simulink model "RobotX_SLAMonly"  (R2014a)
settings: Solver=FixedStepDiscrete  StartTime=0.0  StopTime=inf  FixedStep=.25  RelTol=1e-3
undefined symbols (not defined in the file): Com1, Com2, Com3, Com4, DiscIntNeverNeededParam, standard
libraries: xpcseriallib x11, simulink x3, slrtlib x3, dspmtrx3 x2, speedgoatlib x1, speedgoatlib_IO102 x1
(part 4 of 15)

== matlab function RobotX_SLAMonly/Main FSM/SLAM/Models for prediction/Model43/Non-Holonomic Constraint ==
  data: time input; surgeAccel input; NEyaw output; swayAccel input; YawAccel input; u input; v input; gyrz input; psi input; X input; Y input
function NEyaw  = nonHolonomicNE(time,surgeAccel,swayAccel,YawAccel,u,v,gyrz,psi,X,Y)
%Written by Anderson Lebbad on August 12, 2014
%Last Edited:

%This function estimates the velocities for a new pose based off the 
%velocities and heading calculated from the dynamic model, and the current 
%pose. Uses a non-holonomic constraint for estimation.

%% Find time elapsed for integration

ts = .1;
persistent uPrev vPrev gyrzPrev psiPrev xPrev yPrev

%Initialize
if isempty(uPrev)
    uPrev = [u time];
    vPrev = [v time];
    gyrzPrev = [gyrz time];
    psiPrev = [psi time];
    xPrev = [X time];
    yPrev = [Y time];
end
    
%Update if change
if uPrev(1) ~= u
    uPrev = [u time];
end
if vPrev(1) ~= v
    vPrev = [v time];
end
if gyrzPrev(1) ~= gyrz
    gyrzPrev = [gyrz time];
end
if psiPrev(1) ~= psi
    psiPrev = [psi time];
end
if xPrev(1) ~= X
    xPrev = [X time];
end
if yPrev(1) ~= Y
    yPrev = [Y time];
end

%evaluate elapsed
uTime = ts + time - uPrev(2);
vTime = ts + time - vPrev(2);
gyrzTime = ts + time - gyrzPrev(2);
psiTime = ts + time - psiPrev(2);
xTime = ts + time - xPrev(2);
yTime = ts + time - yPrev(2);

%% Integrate inputs
surgeVel = u + surgeAccel*uTime/2;
swayVel = v + swayAccel*vTime/2;
yawVel = gyrz + YawAccel*gyrzTime/2;
yaw = psi + yawVel*psiTime/2;


%% Apply Non-holonomic constraint for NE velocities
Xd = surgeVel*cos(yaw*pi/180) - swayVel*sin(yaw*pi/180);
Yd = surgeVel*sin(yaw*pi/180) + swayVel*cos(yaw*pi/180);

%% Integrate to output NE coordinates
N = X + Xd*xTime/2;
E = Y + Yd*yTime/2;

NEyaw = [N;E;yaw];

end

== matlab function RobotX_SLAMonly/Main FSM/SLAM/Models for prediction/Model43/move_part ==
  data: PtThrust input; portMP output; PtAzimuth input; StThrust input; StAzimuth input; noiseLevel input; portAzimuth output; stbdMP output; stbdAzimuth output
function [portMP,portAzimuth,stbdMP,stbdAzimuth] = addNoise(PtThrust,...
    PtAzimuth,StThrust,StAzimuth,noiseLevel)
%Written By Anderson Lebbad on September 16, 2014
%Last Edited By:

%This function adds gaussian noise to the inputs for a particular particles
%model

portMP = normrnd(PtThrust, noiseLevel);
portAzimuth = normrnd(PtAzimuth, noiseLevel);
stbdMP = normrnd(StThrust, noiseLevel);
stbdAzimuth = normrnd(StAzimuth, noiseLevel);

end

== matlab function RobotX_SLAMonly/Main FSM/SLAM/Models for prediction/Model44/Dynamic Model ==
  data: F_surge input; F_sway input; Torque input; u input; surgeAccel output; v input; psi input; swayAccel output; yawAccel output
function [surgeAccel, swayAccel, yawAccel] = ...
    WAM_V_3DOF(F_surge, F_sway, Torque, u, v, psi)
%Written by Anderson Lebbad on August 12, 2014
%Last Edited:

%This function was heavily based off of Ariel Qu's Vel3DOF_IvanV1. It was
%rewritten for real-time use.

%This function will produce the transient output surge velocity of a
%linearized model of the USV. It is assumed that the vehicle is equivalent
%to two cylinders in the water.

%%%%%DEFINED VARIABLE%%%%%%
%
%   Xext = Thrust from motors
%   Next = Moment from motor
%   m = Mass of vehicle
%   Xudot = Added mass in surge direction
%   Yvdot = Added mass in sway direction
%   Nrdot = Added mass from yaw
%   xg = offset from center of gravity
%   rho = density of seawater
%   S = wetted surface area
%   R = Reynolds number
%   Cd = Coefficient of drag
%   Cdc = Coefficient of drag for sway
%   nu = Kinematic viscosity
%   L = Length overall
%   T = draft
%   B = beam
%   SA = Surface area of cylinder experiencing sway
%   Iz = moment of inertia about Z axis
%
%%%%%%

% Force/Mometns from thrusters & control surfaces...

tau = [F_surge; F_sway; Torque];

% Calculate yaw rate
persistent lastHeading
if isempty(lastHeading)
    lastHeading = psi;
end
%Sample time
ts = .1;

r = (psi - lastHeading)/ts;

% Velocity & Angular velocity vectors
vel = [u; v; 0];
omega = [0; 0; r];

%define variables
m = 145.7;         % Total mass [kg] - reduced from 102
rho = 1025.9;   % density of seawater [kg/m^3]
L = 3.91*0.85;  % Length on the waterline [m]
B = 0.426;       % Demihull beam [m]
T = B*0.2;        % Draft of the demihull [m]
p_bar = 1.0; % sidehull separation - from centerplane vessel to centerplane demihull
Iz = 262.181;    % Mass moment of inertia about z-axis [kg*m^2]
xg = 0;         % Body-Fixed coordinate system taken to be center of gravity
yg = 0;         % Symmetrical Vessel
Cd = 1.1;       % Drag coefficient for a lateral cylinder
LCG = 1.485;        % Need to know where LCG wrt stern

% Vector location of port and starboard hulls
r_port = [-LCG; -p_bar; 0];   
r_stbd = [-LCG; p_bar; 0];

% Port and starboard hull velocities
vel_port = vel + cross(omega,r_port);
vel_stbd = vel + cross(omega,r_stbd);

u_port = vel_port(1);
u_stbd = vel_stbd(1);

% Port and starboard state vectors
state_port = vel_port + omega;
state_stbd = vel_stbd + omega;

%% Added Mass
% Estimated for each hull, then multiplied by 2 to account for both hulls
Xudot = -0.05*m;

%Using strip theory to estimate added mass coefficients
Nrdot = -(4.75/2*pi*rho*p_bar*T^4 + pi*rho*T^2*((L - LCG)^3 + LCG^3)/3);
Nvdot = - pi*rho*T^2*((L - LCG)^2 - LCG^2)/2;

Yrdot = Nvdot;
Yvdot = -rho*pi*T^2*L;

% Multiply by 2:
Xudot = 2*Xudot;
Nrdot = 2*Nrdot;
Nvdot = 2*Nvdot;
Yrdot = 2*Yrdot;
Yvdot = 2*Yvdot;

%Calculate Coefficient of Drag for Sway from 1950 SNAME approximation
Cdc= 1.1 + 0.0045*L/T - 0.1*B/T + 0.016*(B/T)^2;
SA = 2*pi/4*T*L; %projected area of pontoon for two pontoons

%% Linear Drag Terms
%Total Speed
U = sqrt(u^2+v^2);

Xu = 0;
Yv = -0.5*rho*abs(v)*2*Cdc*SA; %20 was the last working number %from SNAME 1950, x2 for two cylinders
%Nr = -0.5*pi*rho*U*T^2*L^2;
Nr = -pi*rho*U*T^2*L^2*.065;
Nv = -pi*rho*U*T^2*L*.01;
Yr = pi*rho*U*T^2*L*0.2;  %from Newman approximation in Lewandowski

%% Nonlinear Drag Terms

% Drag and Moment due to drag on entire vessel - includes nonlinear and
% linear drag terms
D_port = 0.5*(0.44*u_port^3 - 0.01*u_port^2 + 19*u_port);     % Can assume that this equation also takes into account Xu - so set Xu=0
D_stbd = 0.5*(0.44*u_stbd^3 - 0.01*u_stbd^2 + 19*u_stbd);     % Can assume that this equation also takes into account Xu - so set Xu=0

tau_drag = [-(D_port + D_stbd); 0; (D_stbd - D_port)*p_bar];

Xuu = 0;

%% Maneuvering Coefficient Matrices
% Added Mass Matrix
M = [(m - Xudot)      0              0;...
    0               (m - Yvdot)     (m*xg - Yrdot);...
    0               (m*xg - Nvdot)  (Iz - Nrdot)];

%Centripetal and Added Mass Centripetal force matrices
% C_RB = [
%     0                  0                0
%     0                  0                0
%     0                  0                0
%     ];

% C_RB = [
%     0                  0                -m*(xg*r + v)
%     0                  0                -m*(yg*r - u)
%     m*(xg*r + v)       m*(yg*r - u)     0
%     ];

% C_A = -[ %negative originally
%     0                               0           0
%     0                               0           0
%     0                               0           0
%     ];

% Negating centripetal acceleration for test
C_RB = 0;
C_A = 0;

D = -[Xu  0   0;...
      0   Yv  Yr;...
      0   Nv  Nr];

% Nonlinear Drag Coefficients
D_N = -[Xuu*u   0                       0;...
        0       0                       0;...
        0       0                       0];
    
%% Calculate the port and starboard force vectors
tau_port = -(C_RB + C_A + D + D_N)*state_port;
tau_stbd = -(C_RB + C_A + D + D_N)*state_stbd;


%% Sum the force vectors
tau_tot = tau + tau_drag + tau_port + tau_stbd...
    + cross(r_port,[tau_port(1);tau_port(2);0]) + ...
    cross(r_stbd,[tau_stbd(1);tau_stbd(2);0]);

% Calculate the time derivative of the state vector

accel = M\tau_tot;

%% Separate output

surgeAccel = accel(1);
swayAccel = accel(2);
yawAccel = accel(3);

end

== matlab function RobotX_SLAMonly/Main FSM/SLAM/Models for prediction/Model46/Port Thruster Model ==
  data: portMP input; F_surge output; portAzimuth input; F_sway output; Torque output
function [F_surge,F_sway,Torque]  = PortThruster(portMP,portAzimuth)
%Approximation for Starboard Force and Moment with the input motor power
%and azimuth angle of thruster

%Longitudinal distance from center of mass
longDist =1.007;           %m

%Axial distance from center of mass
axialDist=1.485;            %m

%% Piece-wise thrust calculation

if portMP <= -51.0119
    F = .9140*portMP + 40;
elseif portMP >= 26.8367
    F = 1.658*portMP - 41.01;
else
    F = .12987*portMP;
end

%% Force components
F_surge=F*cos(portAzimuth*pi/180);       %N
F_sway=F*sin(portAzimuth*pi/180);       %N

%% Torque calculation

Torque = F_surge*longDist - F_sway*axialDist;   %N.m

end

== matlab function RobotX_SLAMonly/Main FSM/SLAM/Models for prediction/Model46/Stbd Thruster Model ==
  data: stbdMP input; F_surge output; stbdAzimuth input; F_sway output; Torque output
function [F_surge,F_sway,Torque]  = StarBoardThruster(stbdMP,stbdAzimuth)
%Approximation for Starboard Force and Moment with the input motor power
%and azimuth angle of thruster

%Longitudinal distance from center of mass
longDist =1.007;           %m

%Axial distance from center of mass
axialDist=1.485;            %m

%% Piece-wise thrust calculation

if stbdMP <= -51.0119
    F = .9140*stbdMP + 40;
elseif stbdMP >= 26.8367
    F = 1.658*stbdMP - 41.01;
else
    F = .12987*stbdMP;
end

%% Force components
F_surge=F*cos(stbdAzimuth*pi/180);       %N
F_sway=F*sin(stbdAzimuth*pi/180);       %N

%% Torque calculation

Torque = -F_surge*longDist - F_sway*axialDist;   %N.m

end

== matlab function RobotX_SLAMonly/Main FSM/SLAM/Models for prediction/Model47/Non-Holonomic Constraint ==
  data: time input; surgeAccel input; NEyaw output; swayAccel input; YawAccel input; u input; v input; gyrz input; psi input; X input; Y input
function NEyaw  = nonHolonomicNE(time,surgeAccel,swayAccel,YawAccel,u,v,gyrz,psi,X,Y)
%Written by Anderson Lebbad on August 12, 2014
%Last Edited:

%This function estimates the velocities for a new pose based off the 
%velocities and heading calculated from the dynamic model, and the current 
%pose. Uses a non-holonomic constraint for estimation.

%% Find time elapsed for integration

ts = .1;
persistent uPrev vPrev gyrzPrev psiPrev xPrev yPrev

%Initialize
if isempty(uPrev)
    uPrev = [u time];
    vPrev = [v time];
    gyrzPrev = [gyrz time];
    psiPrev = [psi time];
    xPrev = [X time];
    yPrev = [Y time];
end
    
%Update if change
if uPrev(1) ~= u
    uPrev = [u time];
end
if vPrev(1) ~= v
    vPrev = [v time];
end
if gyrzPrev(1) ~= gyrz
    gyrzPrev = [gyrz time];
end
if psiPrev(1) ~= psi
    psiPrev = [psi time];
end
if xPrev(1) ~= X
    xPrev = [X time];
end
if yPrev(1) ~= Y
    yPrev = [Y time];
end

%evaluate elapsed
uTime = ts + time - uPrev(2);
vTime = ts + time - vPrev(2);
gyrzTime = ts + time - gyrzPrev(2);
psiTime = ts + time - psiPrev(2);
xTime = ts + time - xPrev(2);
yTime = ts + time - yPrev(2);

%% Integrate inputs
surgeVel = u + surgeAccel*uTime/2;
swayVel = v + swayAccel*vTime/2;
yawVel = gyrz + YawAccel*gyrzTime/2;
yaw = psi + yawVel*psiTime/2;


%% Apply Non-holonomic constraint for NE velocities
Xd = surgeVel*cos(yaw*pi/180) - swayVel*sin(yaw*pi/180);
Yd = surgeVel*sin(yaw*pi/180) + swayVel*cos(yaw*pi/180);

%% Integrate to output NE coordinates
N = X + Xd*xTime/2;
E = Y + Yd*yTime/2;

NEyaw = [N;E;yaw];

end

== matlab function RobotX_SLAMonly/Main FSM/SLAM/Models for prediction/Model47/move_part ==
  data: PtThrust input; portMP output; PtAzimuth input; StThrust input; StAzimuth input; noiseLevel input; portAzimuth output; stbdMP output; stbdAzimuth output
function [portMP,portAzimuth,stbdMP,stbdAzimuth] = addNoise(PtThrust,...
    PtAzimuth,StThrust,StAzimuth,noiseLevel)
%Written By Anderson Lebbad on September 16, 2014
%Last Edited By:

%This function adds gaussian noise to the inputs for a particular particles
%model

portMP = normrnd(PtThrust, noiseLevel);
portAzimuth = normrnd(PtAzimuth, noiseLevel);
stbdMP = normrnd(StThrust, noiseLevel);
stbdAzimuth = normrnd(StAzimuth, noiseLevel);

end

== matlab function RobotX_SLAMonly/Main FSM/SLAM/Models for prediction/Model48/Dynamic Model ==
  data: F_surge input; F_sway input; Torque input; u input; surgeAccel output; v input; psi input; swayAccel output; yawAccel output
function [surgeAccel, swayAccel, yawAccel] = ...
    WAM_V_3DOF(F_surge, F_sway, Torque, u, v, psi)
%Written by Anderson Lebbad on August 12, 2014
%Last Edited:

%This function was heavily based off of Ariel Qu's Vel3DOF_IvanV1. It was
%rewritten for real-time use.

%This function will produce the transient output surge velocity of a
%linearized model of the USV. It is assumed that the vehicle is equivalent
%to two cylinders in the water.

%%%%%DEFINED VARIABLE%%%%%%
%
%   Xext = Thrust from motors
%   Next = Moment from motor
%   m = Mass of vehicle
%   Xudot = Added mass in surge direction
%   Yvdot = Added mass in sway direction
%   Nrdot = Added mass from yaw
%   xg = offset from center of gravity
%   rho = density of seawater
%   S = wetted surface area
%   R = Reynolds number
%   Cd = Coefficient of drag
%   Cdc = Coefficient of drag for sway
%   nu = Kinematic viscosity
%   L = Length overall
%   T = draft
%   B = beam
%   SA = Surface area of cylinder experiencing sway
%   Iz = moment of inertia about Z axis
%
%%%%%%

% Force/Mometns from thrusters & control surfaces...

tau = [F_surge; F_sway; Torque];

% Calculate yaw rate
persistent lastHeading
if isempty(lastHeading)
    lastHeading = psi;
end
%Sample time
ts = .1;

r = (psi - lastHeading)/ts;

% Velocity & Angular velocity vectors
vel = [u; v; 0];
omega = [0; 0; r];

%define variables
m = 145.7;         % Total mass [kg] - reduced from 102
rho = 1025.9;   % density of seawater [kg/m^3]
L = 3.91*0.85;  % Length on the waterline [m]
B = 0.426;       % Demihull beam [m]
T = B*0.2;        % Draft of the demihull [m]
p_bar = 1.0; % sidehull separation - from centerplane vessel to centerplane demihull
Iz = 262.181;    % Mass moment of inertia about z-axis [kg*m^2]
xg = 0;         % Body-Fixed coordinate system taken to be center of gravity
yg = 0;         % Symmetrical Vessel
Cd = 1.1;       % Drag coefficient for a lateral cylinder
LCG = 1.485;        % Need to know where LCG wrt stern

% Vector location of port and starboard hulls
r_port = [-LCG; -p_bar; 0];   
r_stbd = [-LCG; p_bar; 0];

% Port and starboard hull velocities
vel_port = vel + cross(omega,r_port);
vel_stbd = vel + cross(omega,r_stbd);

u_port = vel_port(1);
u_stbd = vel_stbd(1);

% Port and starboard state vectors
state_port = vel_port + omega;
state_stbd = vel_stbd + omega;

%% Added Mass
% Estimated for each hull, then multiplied by 2 to account for both hulls
Xudot = -0.05*m;

%Using strip theory to estimate added mass coefficients
Nrdot = -(4.75/2*pi*rho*p_bar*T^4 + pi*rho*T^2*((L - LCG)^3 + LCG^3)/3);
Nvdot = - pi*rho*T^2*((L - LCG)^2 - LCG^2)/2;

Yrdot = Nvdot;
Yvdot = -rho*pi*T^2*L;

% Multiply by 2:
Xudot = 2*Xudot;
Nrdot = 2*Nrdot;
Nvdot = 2*Nvdot;
Yrdot = 2*Yrdot;
Yvdot = 2*Yvdot;

%Calculate Coefficient of Drag for Sway from 1950 SNAME approximation
Cdc= 1.1 + 0.0045*L/T - 0.1*B/T + 0.016*(B/T)^2;
SA = 2*pi/4*T*L; %projected area of pontoon for two pontoons

%% Linear Drag Terms
%Total Speed
U = sqrt(u^2+v^2);

Xu = 0;
Yv = -0.5*rho*abs(v)*2*Cdc*SA; %20 was the last working number %from SNAME 1950, x2 for two cylinders
%Nr = -0.5*pi*rho*U*T^2*L^2;
Nr = -pi*rho*U*T^2*L^2*.065;
Nv = -pi*rho*U*T^2*L*.01;
Yr = pi*rho*U*T^2*L*0.2;  %from Newman approximation in Lewandowski

%% Nonlinear Drag Terms

% Drag and Moment due to drag on entire vessel - includes nonlinear and
% linear drag terms
D_port = 0.5*(0.44*u_port^3 - 0.01*u_port^2 + 19*u_port);     % Can assume that this equation also takes into account Xu - so set Xu=0
D_stbd = 0.5*(0.44*u_stbd^3 - 0.01*u_stbd^2 + 19*u_stbd);     % Can assume that this equation also takes into account Xu - so set Xu=0

tau_drag = [-(D_port + D_stbd); 0; (D_stbd - D_port)*p_bar];

Xuu = 0;

%% Maneuvering Coefficient Matrices
% Added Mass Matrix
M = [(m - Xudot)      0              0;...
    0               (m - Yvdot)     (m*xg - Yrdot);...
    0               (m*xg - Nvdot)  (Iz - Nrdot)];

%Centripetal and Added Mass Centripetal force matrices
% C_RB = [
%     0                  0                0
%     0                  0                0
%     0                  0                0
%     ];

% C_RB = [
%     0                  0                -m*(xg*r + v)
%     0                  0                -m*(yg*r - u)
%     m*(xg*r + v)       m*(yg*r - u)     0
%     ];

% C_A = -[ %negative originally
%     0                               0           0
%     0                               0           0
%     0                               0           0
%     ];

% Negating centripetal acceleration for test
C_RB = 0;
C_A = 0;

D = -[Xu  0   0;...
      0   Yv  Yr;...
      0   Nv  Nr];

% Nonlinear Drag Coefficients
D_N = -[Xuu*u   0                       0;...
        0       0                       0;...
        0       0                       0];
    
%% Calculate the port and starboard force vectors
tau_port = -(C_RB + C_A + D + D_N)*state_port;
tau_stbd = -(C_RB + C_A + D + D_N)*state_stbd;


%% Sum the force vectors
tau_tot = tau + tau_drag + tau_port + tau_stbd...
    + cross(r_port,[tau_port(1);tau_port(2);0]) + ...
    cross(r_stbd,[tau_stbd(1);tau_stbd(2);0]);

% Calculate the time derivative of the state vector

accel = M\tau_tot;

%% Separate output

surgeAccel = accel(1);
swayAccel = accel(2);
yawAccel = accel(3);

end

== matlab function RobotX_SLAMonly/Main FSM/SLAM/Models for prediction/Model50/Port Thruster Model ==
  data: portMP input; F_surge output; portAzimuth input; F_sway output; Torque output
function [F_surge,F_sway,Torque]  = PortThruster(portMP,portAzimuth)
%Approximation for Starboard Force and Moment with the input motor power
%and azimuth angle of thruster

%Longitudinal distance from center of mass
longDist =1.007;           %m

%Axial distance from center of mass
axialDist=1.485;            %m

%% Piece-wise thrust calculation

if portMP <= -51.0119
    F = .9140*portMP + 40;
elseif portMP >= 26.8367
    F = 1.658*portMP - 41.01;
else
    F = .12987*portMP;
end

%% Force components
F_surge=F*cos(portAzimuth*pi/180);       %N
F_sway=F*sin(portAzimuth*pi/180);       %N

%% Torque calculation

Torque = F_surge*longDist - F_sway*axialDist;   %N.m

end

== matlab function RobotX_SLAMonly/Main FSM/SLAM/Models for prediction/Model50/Stbd Thruster Model ==
  data: stbdMP input; F_surge output; stbdAzimuth input; F_sway output; Torque output
function [F_surge,F_sway,Torque]  = StarBoardThruster(stbdMP,stbdAzimuth)
%Approximation for Starboard Force and Moment with the input motor power
%and azimuth angle of thruster

%Longitudinal distance from center of mass
longDist =1.007;           %m

%Axial distance from center of mass
axialDist=1.485;            %m

%% Piece-wise thrust calculation

if stbdMP <= -51.0119
    F = .9140*stbdMP + 40;
elseif stbdMP >= 26.8367
    F = 1.658*stbdMP - 41.01;
else
    F = .12987*stbdMP;
end

%% Force components
F_surge=F*cos(stbdAzimuth*pi/180);       %N
F_sway=F*sin(stbdAzimuth*pi/180);       %N

%% Torque calculation

Torque = -F_surge*longDist - F_sway*axialDist;   %N.m

end

== matlab function RobotX_SLAMonly/Main FSM/SLAM/Landmark Organizer ==
  data: Distances input; lm_data output; Angles input
function lm_data = lmOrganize(Distances,Angles)
%Written By Anderson Lebbad on September 16, 2014
%Last Edited by:

%This function structures the landmark data to be used for the SLAM

landmarks = [0.01*Distances'; pi/180*Angles'];
[M,N] = size(landmarks);
lm_data = landmarks(1:M*N);

end

== matlab function RobotX_SLAMonly/Main FSM/SLAM/Any State Change ==
  data: u input; y output
function y = fcn(u)
%#codegen

y = any(any(u));

end

== matlab function RobotX_SLAMonly/Main FSM/SLAM/Any Landmark Change ==
  data: u input; y output
function y = fcn(u)
%#codegen

y = any(any(u));

end

== matlab function RobotX_SLAMonly/Main FSM/SLAM/Models for prediction/Model1/Non-Holonomic Constraint ==
  data: time input; surgeAccel input; NEyaw output; swayAccel input; YawAccel input; u input; v input; gyrz input; psi input; X input; Y input
function NEyaw  = nonHolonomicNE(time,surgeAccel,swayAccel,YawAccel,u,v,gyrz,psi,X,Y)
%Written by Anderson Lebbad on August 12, 2014
%Last Edited:

%This function estimates the velocities for a new pose based off the 
%velocities and heading calculated from the dynamic model, and the current 
%pose. Uses a non-holonomic constraint for estimation.

%% Find time elapsed for integration

ts = .1;
persistent uPrev vPrev gyrzPrev psiPrev xPrev yPrev

%Initialize
if isempty(uPrev)
    uPrev = [u time];
    vPrev = [v time];
    gyrzPrev = [gyrz time];
    psiPrev = [psi time];
    xPrev = [X time];
    yPrev = [Y time];
end
    
%Update if change
if uPrev(1) ~= u
    uPrev = [u time];
end
if vPrev(1) ~= v
    vPrev = [v time];
end
if gyrzPrev(1) ~= gyrz
    gyrzPrev = [gyrz time];
end
if psiPrev(1) ~= psi
    psiPrev = [psi time];
end
if xPrev(1) ~= X
    xPrev = [X time];
end
if yPrev(1) ~= Y
    yPrev = [Y time];
end

%evaluate elapsed
uTime = ts + time - uPrev(2);
vTime = ts + time - vPrev(2);
gyrzTime = ts + time - gyrzPrev(2);
psiTime = ts + time - psiPrev(2);
xTime = ts + time - xPrev(2);
yTime = ts + time - yPrev(2);

%% Integrate inputs
surgeVel = u + surgeAccel*uTime/2;
swayVel = v + swayAccel*vTime/2;
yawVel = gyrz + YawAccel*gyrzTime/2;
yaw = psi + yawVel*psiTime/2;


%% Apply Non-holonomic constraint for NE velocities
Xd = surgeVel*cos(yaw*pi/180) - swayVel*sin(yaw*pi/180);
Yd = surgeVel*sin(yaw*pi/180) + swayVel*cos(yaw*pi/180);

%% Integrate to output NE coordinates
N = X + Xd*xTime/2;
E = Y + Yd*yTime/2;

NEyaw = [N;E;yaw];

end

== matlab function RobotX_SLAMonly/Main FSM/SLAM/SLAM enabled/slammed ==
  data: mpa output; lm_data input; pre_part_positions input; part_positions output
%% SLAM by Chidananda Matada Shivananda
%  Copyright 2010 Randolph Voorhies

%  Edited 2014 Nick DiLeo - Modifications for unknown data association
%  and multiple measurements in a single timestep

%  Edited 2014 Chidananda Matada Shivananda - Simulink compatability, New
%  clustering technique added

%  This program is free software: you can redistribute it and/or modify
%  it under the terms of the GNU General Public License as published by
%  the Free Software Foundation, either version 3 of the License, or
%  (at your option) any later version.
%
%  This program is distributed in the hope that it will be useful,
%  but WITHOUT ANY WARRANTY; without even the implied warranty of
%  MERCHANTABILITY or FITNESS FOR A PARTICULAR PURPOSE.  See the
%  GNU General Public License for more details.
%
%  You should have received a copy of the GNU General Public License
%  along with this program.  If not, see <http://www.gnu.org/licenses/>.

function [mpa,part_positions]   = slammed(lm_data,pre_part_positions)

%% General comments

% the angles in radians
% the ditance in m



%% Initialisations.

persistent particles avg_robot;
num_particles = 50;

% the limits
max_read_distance = 20;
min_read_distance = 0.3;
min_read_angle = -60*pi/180; %radians- maximum read angle
max_read_angle = 60*pi/180;

% The initial starting position of the robot Use UTM coordinates from GPS
avg_robot_position = [0;0;0];% x y rotation

% The Gaussian variance of the movement commands
% Approximating there are only two drives
% movement_variance = [.1;.1];   % Left drive Right_drive
% M = [movement_variance(1), 0.0;
%      0.0, movement_variance(2)];
measurement_variance = [0.01; 0.01];   % Distance Angle
R = [measurement_variance(1), 0.0;
    0.0, measurement_variance(2)];

default_importance=0.00000000001;

if isempty(particles)
    %  Particles
    %             w[1]
    %             position[1,3]
    %             num_landmarks[300] this is to keep history
    
    %             lm_weight[2,15]based on number of landmarks
    %             landmarks[15]
    %                         position[2,1]
    %                         E[2,2]
    %                         counter[1]
    particles=repmat(struct('w',1.0/num_particles,'position',avg_robot_position,'num_landmarks',zeros(1,2),'lm_weight',repmat(1.0/num_particles,2,15),'landmarks',repmat(struct('pos',zeros(1,2),'E',zeros(2,2),'counter',0),1,15)),1,50);
    avg_robot_position = average_pos(particles,num_particles);
end

if isempty(avg_robot)
    avg_robot=avg_robot_position;
end


avg_robot_position=avg_robot;

%% Upload the moved data onto the particles
for shiva9=1:50
    particles(shiva9).position(1)= pre_part_positions(3*(shiva9-1)+1);
    particles(shiva9).position(2)= pre_part_positions(3*(shiva9-1)+1);
    particles(shiva9).position(3)= pre_part_positions(3*(shiva9-1)+1);
end

%% Try to take a reading from each landmark and calculate the Jacobian
doResample = false;
% The input got from landmarks
[~,cols]=find(lm_data ~= 0);
if (isempty(cols)==0)% if the cols is not empty
    doResample=true; %if there is new measurement, then resample particles
end

if (doResample==true)
    [r,~]=size(cols);
    shiva=1;
    G=zeros(2,2,ceil(r/2));
    z_real=zeros(2,ceil(r/2));
    read_distance=zeros(ceil(r/2));
    read_angle=zeros(ceil(r/2));
    
    for lIdx = 1:2:r %amount of visible landmarks
        real_landmark = [lm_data(cols(lIdx+1)),lm_data(cols(lIdx))];
        % Take a real (noisy) measurement from the robot to the landmark
        %         [z_real(:,lIdx), G(:,:,lIdx)] = getRealMeasurement(avg_robot_position, real_landmark, [0 0]);
        %         function [z, H] = getRealMeasurement(pos, landmark_pos, observation_variance)
        
        landmark_angle=real_landmark(1);
        landmark_distance=real_landmark(2);
        % Compute the Jacobian of this measurement function
        q = landmark_distance^2.0;
        G(:,:,shiva) = [-(real_landmark(1) - avg_robot_position(1))/sqrt(q), -(real_landmark(2) - avg_robot_position(2))/sqrt(q);
            (real_landmark(2) - avg_robot_position(2))/q,       -(real_landmark(1) - avg_robot_position(1))/q];
        
        z_real(:,shiva) = [landmark_distance; landmark_angle];
        read_distance(shiva) = z_real(1,shiva);
        read_angle(shiva)    = z_real(2,shiva);
        shiva=shiva+1;
    end
    %     shiva=1;
    
    for pIdx = 1:num_particles
        %     particles(pIdx).lm_weight=[];
        %     clear z_p H Q
        %         coder.varsize('H', [2,2,16],[0 0 1]);
        num_landmarks=particles(pIdx).num_landmarks(1);
        assert(num_landmarks<20);
        H=zeros(2,2,num_landmarks);
        %         coder.varsize('z_p', [2 1 16]);
        z_p=zeros(2,1,num_landmarks);
        Q=zeros(2,2,num_landmarks);
        for j=1:particles(pIdx).num_landmarks(1)
            %             [z_p(:,j), H(:,:,j)] = getMeasurement(particles(pIdx).position, particles(pIdx).landmarks(j).pos, [0 0]);
            %             function [z, H] = getRealMeasurement(pos, landmark_pos, observation_variance)
            landmark_angle=particles(pIdx).landmarks(j).pos(1);
            landmark_distance=particles(pIdx).landmarks(j).pos(2);
            
            % Compute the Jacobian of this measurement function
            q = landmark_distance^2.0;
            %   H = [-(landmark_pos(1) - pos(1))/sqrt(q), -(landmark_pos(2) - pos(2))/sqrt(q), 0.0;
            %         (landmark_pos(2) - pos(2))/q,       -(landmark_pos(1) - pos(1))/q,      -1.0;
            %         0.0,                                0.0,                               1.0];
            
            H(:,:,j) = [-(particles(pIdx).landmarks(j).pos(1) - particles(pIdx).position(1))/sqrt(q), -(particles(pIdx).landmarks(j).pos(2) - particles(pIdx).position(2))/sqrt(q);
                (particles(pIdx).landmarks(j).pos(2) - particles(pIdx).position(2))/q,       -(particles(pIdx).landmarks(j).pos(1) - particles(pIdx).position(1))/q];
            
            
            z_p(:,j) = [landmark_distance;
                landmark_angle];
            
            for measured_lm=1:size(z_real,2)
                residual = z_real(:,measured_lm) - z_p(:,j);
                Q(:,:,j) = H(:,:,j)' * particles(pIdx).landmarks(j).E * H(:,:,j) + R;
                particles(pIdx).lm_weight(measured_lm,j) = particles(pIdx).w * norm(2*pi*Q(:,:,j)).^(-1/2)*exp(-1/2*(residual'/Q(:,:,j)*residual));
            end
        end
        
        particles(pIdx).num_landmarks(2)=particles(pIdx).num_landmarks(1);
        num_landmarks2=particles(pIdx).num_landmarks(2);
        assert(num_landmarks2<20);
        
        %           clear c_hat
        %         clear cost_table data_associate_mat data_associate_vect
        %%%%%%%%%%%%%%%%%%%%%%%%%%%%%%%%%%%%%%%%%%%%%%%%%%%%%%%%%%%%%%%%%%%%%%%%%%%%%%%%%%%%%%%%%%%%%%%%%%%%%%%%%%%%%%%%%%%%%%%%%%%%%%%%%%%%%%%%%%%%%
        cost_table=zeros(size(z_real,2),num_landmarks+size(z_real,2));
        %         cost_table=zeros(size(z_real,2),num_landmarks);
        cost_table(1:size(z_real,2),1:particles(pIdx).num_landmarks(1))=particles(pIdx).lm_weight(1:size(z_real,2),1:particles(pIdx).num_landmarks(1));
        cost_table(1:size(z_real,2),particles(pIdx).num_landmarks(1)+1:particles(pIdx).num_landmarks(1)+size(z_real,2)) =default_importance*eye(size(z_real,2));
        
        particles(pIdx).w=max(max(cost_table,[],1),[],2);
        [~, idx_hold]=max(cost_table,[],1); %this is the max correseponding for each measurement
        for i=1:size(cost_table,2)
            idx_zero=setdiff(1:size(cost_table,1),idx_hold(i));
            cost_table(idx_zero,i)=0;
        end
        
        cost_table1=cost_table;
        for shiva14=1:size(cost_table,2)
            cost_table(:,shiva14)=cost_table1(:,size(cost_table,2)-shiva14+1);
        end
        
        
        new_landmarks=0;
        for measured_lm=1:size(z_real,2)
            [~, IDX] = max(cost_table(measured_lm,:));
            if IDX > particles(pIdx).num_landmarks(1)
                new_landmarks=new_landmarks+1;
            end
        end
        
        
        assert(new_landmarks<20);
        data_associate_mat=zeros(size(z_real,2),new_landmarks+num_landmarks2);
        
        for measured_lm=1:size(z_real,2)
            [~, IDX] = max(cost_table(measured_lm,:));
            if IDX > particles(pIdx).num_landmarks(1)
                %we haven't seen this landmark before
                %                 if particles(pIdx).num_landmarks(2)>14
                %                     break;
                %                 end
                particles(pIdx).num_landmarks(2)=particles(pIdx).num_landmarks(2)+1; %add new landmark
                data_associate_mat(measured_lm,particles(pIdx).num_landmarks(2))=measured_lm; %set correspondance b/t measurement and feature j
            else
                %we've already seen this landmark
                %           [val idx]=max(particles(pIdx).lm_weight(measured_lm,:));
                data_associate_mat(measured_lm,IDX)=measured_lm; %measurement is a known feature
            end
            
        end
        
        num_landmarks2=particles(pIdx).num_landmarks(2);
        assert(num_landmarks2<20);
        Hn=zeros(2,2,num_landmarks2);
        t=size(H);
        for i=1:t(3)
            Hn(:,:,i)=H(:,:,i);
        end
        
        %         H=zeros(2,2,num_landmarks2);
        H=Hn;
        
        data_associate_vect=max(data_associate_mat,[],1); %vector that contains measurement correspondance to landmarks
        i=1;
        feature_to_delete=zeros(num_landmarks2);
        for j=1:particles(pIdx).num_landmarks(2) %length(data_associate_vect)
            if (data_associate_vect(j)>0 && j>particles(pIdx).num_landmarks(1))
                % If we have never seen this landmark, then we need to initialize it.
                % We'll just use whatever first reading we recieved.
                particles(pIdx).landmarks(j).pos = [particles(pIdx).position(1) + ...
                    sin(read_angle(data_associate_vect(j))+particles(pIdx).position(3))*read_distance(data_associate_vect(j));...
                    particles(pIdx).position(2) + cos(read_angle(data_associate_vect(j))+particles(pIdx).position(3))*read_distance(data_associate_vect(j))]';
                % Initialize the landmark position covariance
                H(:,:,j)=G(:,:,data_associate_vect(j));
                particles(pIdx).landmarks(j).E = inv(G(:,:,data_associate_vect(j)))' * R * inv(G(:,:,data_associate_vect(j)));
                particles(pIdx).landmarks(j).counter=1; %initialize counter
            elseif (data_associate_vect(j)>0 && j<=particles(pIdx).num_landmarks(1))
                %we've seen this landmark before
                K = particles(pIdx).landmarks(j).E * H(:,:,j) / Q(:,:,j);
                % Mix the ideal reading, and our actual reading using the Kalman gain, and use the result
                % to predict a new landmark position
                particles(pIdx).landmarks(j).pos = particles(pIdx).landmarks(j).pos + (K*(z_real(:,data_associate_vect(j))-z_p(:,j)))';
                % Update the covariance of this landmark
                particles(pIdx).landmarks(j).E = (eye(size(H(:,:,j))) - K*H(:,:,j)')*particles(pIdx).landmarks(j).E;
                particles(pIdx).landmarks(j).counter=particles(pIdx).landmarks(j).counter+1; %increment counter
            else
                % We are leaving these unchanged.  These are commented
                % out, but this is what is actually happening in alg.
                % particles(pIdx).landmarks(j).pos = particles(pIdx).landmarks(j).pos;
                % particles(pIdx).landmarks(j).E=particles(pIdx).landmarks(j).E;
                dist_to_landmark=norm([particles(pIdx).landmarks(j).pos(1)-particles(pIdx).position(1) particles(pIdx).landmarks(j).pos(2)-particles(pIdx).position(2)]);
                ang_to_landmark=atan2((particles(pIdx).landmarks(j).pos(1) - particles(pIdx).position(1)),...
                    (particles(pIdx).landmarks(j).pos(2) - particles(pIdx).position(2)))-particles(pIdx).position(3);
                if (dist_to_landmark > max_read_distance ||dist_to_landmark < min_read_distance || ang_to_landmark > max_read_angle || ang_to_landmark < min_read_angle)
                    %counter(pIdx,j)=counter(pIdx,j) %don't change counter
                else
                    particles(pIdx).landmarks(j).counter=particles(pIdx).landmarks(j).counter-1; %decrement counter
                    if particles(pIdx).landmarks(j).counter<0
                        feature_to_delete(i)=j; %we're going to delete all these features at the end of the loop
                        i=i+1;
                    end
                end
                %
            end %if
        end %end j
        %     'pos',zeros(1,2),'E',zeros(2,2),'counter',0
        if~(isempty(nonzeros(feature_to_delete)))
            tobe_del=nonzeros(feature_to_delete);
            for shiva4=1:length(feature_to_delete)
                particles(pIdx).landmarks(tobe_del(shiva4)).pos=zeros(1,2);
                particles(pIdx).landmarks(tobe_del(shiva4)).E=zeros(2,2);
                particles(pIdx).landmarks(tobe_del(shiva4)).counter=0;
            end
            particles(pIdx).num_landmarks(2)= particles(pIdx).num_landmarks(2)-length(tobe_del);
        end
        
        particles(pIdx).num_landmarks(1)=particles(pIdx).num_landmarks(2);
        
    end %pIdx
    
    particles=resample(particles) ;
    
    
    
end% if (doResample==true)


%% Clustering
landmarks_positions=zeros(15*50,2);
row_counter=0;
for pIdx=1:num_particles
    for j=1:15 %this should be index timestep when in full script
        row_counter=row_counter+1;
        landmarks_positions(row_counter,:)=particles(pIdx).landmarks(j).pos(1:2)';
    end
end

mpa=cluster(landmarks_positions);


%% Final changes to be persistent
avg_robot=avg_robot_position;
part_positions=zeros(150,1);

for shiva9=1:3:150
    part_positions(shiva9)=particles(ceil(shiva9/3)).position(1);
    part_positions(shiva9+1)=particles(ceil(shiva9/3)).position(2);
    part_positions(shiva9+2)=particles(ceil(shiva9/3)).position(3);
end

%% Display and output

end %function [y,y1]  = slammed(imu_data,lm_data)

function [map]= cluster(data)

n=size(data,1);
clusters=ones(n,1);
hubs=zeros(n,1);
hubs(1,1)=1;
dif=zeros(n,2);
% clustersort=zeros(n,3);
for i = 1:n
    dif(i,:)= data(clusters(i),:) - data(i,:);
end
dist =sum((dif.*dif),2);
counter =1;             %Keeps track of number of the present number of hubs
continue12 = 1;   % 1=true 0=false indicates whether to continue forming new

while continue12
    counter = counter + 1;    % adding new hub
    if counter>750
        break;
    end
    [~,i]=max(dist);        %m= maximum value in the distance array
    %i is the location of the maximum value in the
    % array
    hubs(counter)=i;        %assigns index to new hub
    temp = i*ones(n,1);
    dif1=zeros(n,2);
    for i23 = 1:n
        dif1(i23,:)= data(temp(i23),:) - data(i23,:);
    end
    newdist =sum((dif1.*dif1),2);
    for r=1:n
        if newdist(r) < dist(r)
            dist(r)=newdist(r);
            clusters(r)=i;
        end     %end for if
    end
    maxdist=max(dist);      %returns distance of point farthest from its hub
    continue12 = farout(counter,hubs,data,maxdist); %Checks the stop condition
end
clustersort=[data,clusters];
clustersort=sortrows(clustersort,3);
map=zeros(12,2);
temp=zeros(12,1);
temp(1,1)=clustersort(1,3);
shiva12=1;
for i=1:n
    if sum(temp==clustersort(i,3)) == 0
        shiva12=shiva12+1;
        if shiva12>12
            break
        end
        temp(shiva12)=clustersort(i,3);
    end
end
for shiva13=1:12
    clusterIdx = clustersort(:,3)==temp(shiva13);
    map(shiva13,:)=[sum(clustersort(clusterIdx,1)),sum(clustersort(clusterIdx,2))*180/pi]/sum(clusterIdx);
end
end



function continue1 = farout(counter1,hubs1,data1,maxdist1)

%FAROUT continue = farout(counter,hubs,data,maxdist)
%       Calculates stop condition.  Stops if the point farthest from its
%       hub is within the average distance value.

index1 = 0;
n=size(data1,1);
dif=zeros(n,2);
for i1 = 1:(counter1-1)
    for j = i1+1 : counter1
        index1 = index1 + 1;
        if index1>750
            break
        end
        dif(index1,:)=data1(hubs1(i1),:) - data1(hubs1(j),:);
    end
end

dist=sqrt(sum((dif.*dif),2));
average_dist = sum(dist)/(2*index1);
if sqrt(maxdist1) < average_dist/4
    continue1 = 0;
else continue1 =1;
end
end                             % end for farout

function avg_robot_position = average_pos(particles,num_particles)
xsiva=0;
ysiva=0;
rotasiva=0;

for siva=1:num_particles
    xsiva=xsiva+particles(siva).position(1);
    ysiva=ysiva+particles(siva).position(2);
    rotasiva=rotasiva+particles(siva).position(3);
end

avg_robot_position = [xsiva/num_particles; ysiva/num_particles; rotasiva/num_particles];

end

function [newParticles] = resample(oldParticles)
% Resample a group of particles such that those with higher weights have a
% higher chance of being replicated, and those with low weights have a high
% chance of disappearing
num_particles=50;
avg_robot_position = [0;0;0];% x y rotation
newParticles=repmat(struct('w',1.0/num_particles,'position',avg_robot_position,'num_landmarks',zeros(1,2),'lm_weight',repmat(1.0/num_particles,2,15),'landmarks',repmat(struct('pos',zeros(1,2),'E',zeros(2,2),'counter',0),1,15)),1,50);

weightSum = 0;
for i=1:length(oldParticles)
    weightSum = weightSum + oldParticles(i).w;
end
for i=1:length(oldParticles)
    oldParticles(i).w = oldParticles(i).w/weightSum;
end
M = length(oldParticles);
%   newParticles = [];
r = rand / M;
c = oldParticles(1).w;
i = 1;
shiva6=1;
assert(shiva6<51);
for m=1:M
    U = r + (m-1) * M^(-1);
    while U > c
        i = i+1;
        c = c+oldParticles(i).w;
    end
    newParticles(shiva6) = oldParticles(i);
    shiva6=shiva6+1;
end
for i=1:length(newParticles)
    newParticles(i).w = 1.0/length(newParticles);
end
end

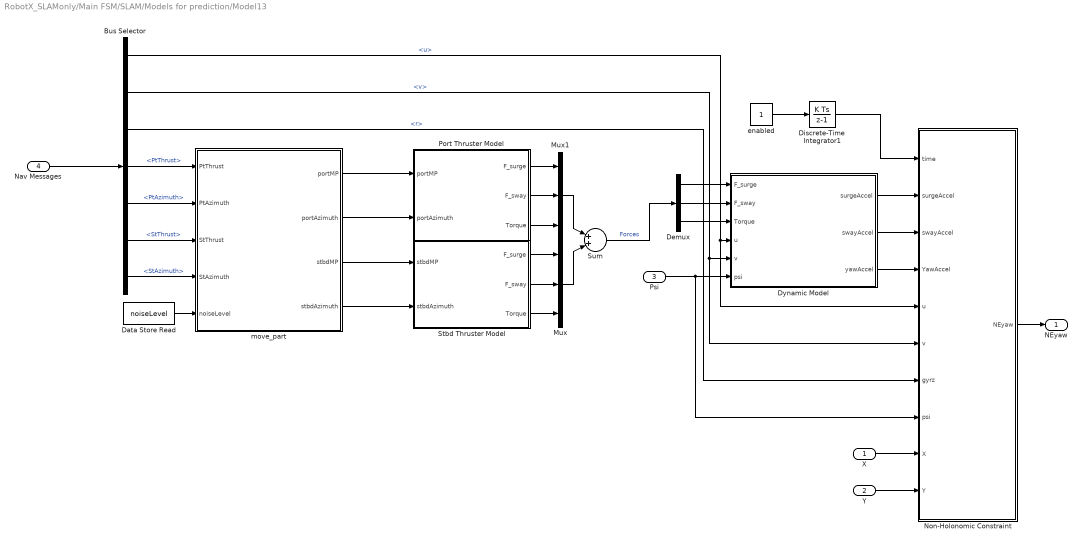
== system RobotX_SLAMonly/Main FSM/SLAM/Models for prediction/Model13 ==
  X : Inport
  Y : Inport  Port=2
  Psi : Inport  Port=3
  Nav Messages : Inport  Port=4
  Bus Selector : BusSelector  OutputSignals=Velocity.u,Velocity.v,Velocity.r,Port.PtThrust,Port.PtAzimuth,Stbd.StThrust,Stbd.StAzimuth
  Data Store Read : DataStoreRead  DataStoreName=noiseLevel
  Demux : Demux  Outputs=3
  Discrete-Time Integrator1 : DiscreteIntegrator  SampleTime=-1  ICPrevOutput=DiscIntNeverNeededParam  ICPrevScaledInput=DiscIntNeverNeededParam
  Dynamic Model : MATLAB Function  TreatAsAtomicUnit=on
  Mux : Mux  Inputs=3
  Mux1 : Mux  Inputs=3
  Non-Holonomic Constraint : MATLAB Function  TreatAsAtomicUnit=on
  Port Thruster Model : MATLAB Function  TreatAsAtomicUnit=on
  Stbd Thruster Model : MATLAB Function  TreatAsAtomicUnit=on
  Sum : Sum  Inputs=|++|
  enabled : Constant
  move_part : MATLAB Function  TreatAsAtomicUnit=on
  NEyaw : Outport
  wires:
  Sum/1 -> Demux/1  "Forces"
  Bus Selector/2 -> Non-Holonomic Constraint/6(v), Dynamic Model/5(v)  "<v>"
  Bus Selector/1 -> Non-Holonomic Constraint/5(u), Dynamic Model/4(u)  "<u>"
  Psi/1 -> Non-Holonomic Constraint/8(psi), Dynamic Model/6(psi)
  Demux/2 -> Dynamic Model/2(F_sway)
  Demux/3 -> Dynamic Model/3(Torque)
  Demux/1 -> Dynamic Model/1(F_surge)
  Mux/1 -> Sum/2
  Stbd Thruster Model/1(F_surge) -> Mux/1
  Stbd Thruster Model/3(Torque) -> Mux/3
  Stbd Thruster Model/2(F_sway) -> Mux/2
  Mux1/1 -> Sum/1
  Port Thruster Model/2(F_sway) -> Mux1/2
  Port Thruster Model/1(F_surge) -> Mux1/1
  Port Thruster Model/3(Torque) -> Mux1/3
  Dynamic Model/1(surgeAccel) -> Non-Holonomic Constraint/2(surgeAccel)
  Dynamic Model/2(swayAccel) -> Non-Holonomic Constraint/3(swayAccel)
  Dynamic Model/3(yawAccel) -> Non-Holonomic Constraint/4(YawAccel)
  Y/1 -> Non-Holonomic Constraint/10(Y)
  X/1 -> Non-Holonomic Constraint/9(X)
  Bus Selector/3 -> Non-Holonomic Constraint/7(gyrz)  "<r>"
  Non-Holonomic Constraint/1(NEyaw) -> NEyaw/1
  enabled/1 -> Discrete-Time Integrator1/1
  Discrete-Time Integrator1/1 -> Non-Holonomic Constraint/1(time)
  Nav Messages/1 -> Bus Selector/1
  Bus Selector/4 -> move_part/1(PtThrust)  "<PtThrust>"
  Bus Selector/5 -> move_part/2(PtAzimuth)  "<PtAzimuth>"
  Bus Selector/7 -> move_part/4(StAzimuth)  "<StAzimuth>"
  Bus Selector/6 -> move_part/3(StThrust)  "<StThrust>"
  move_part/1(portMP) -> Port Thruster Model/1(portMP)
  move_part/2(portAzimuth) -> Port Thruster Model/2(portAzimuth)
  move_part/3(stbdMP) -> Stbd Thruster Model/1(stbdMP)
  move_part/4(stbdAzimuth) -> Stbd Thruster Model/2(stbdAzimuth)
  Data Store Read/1 -> move_part/5(noiseLevel)

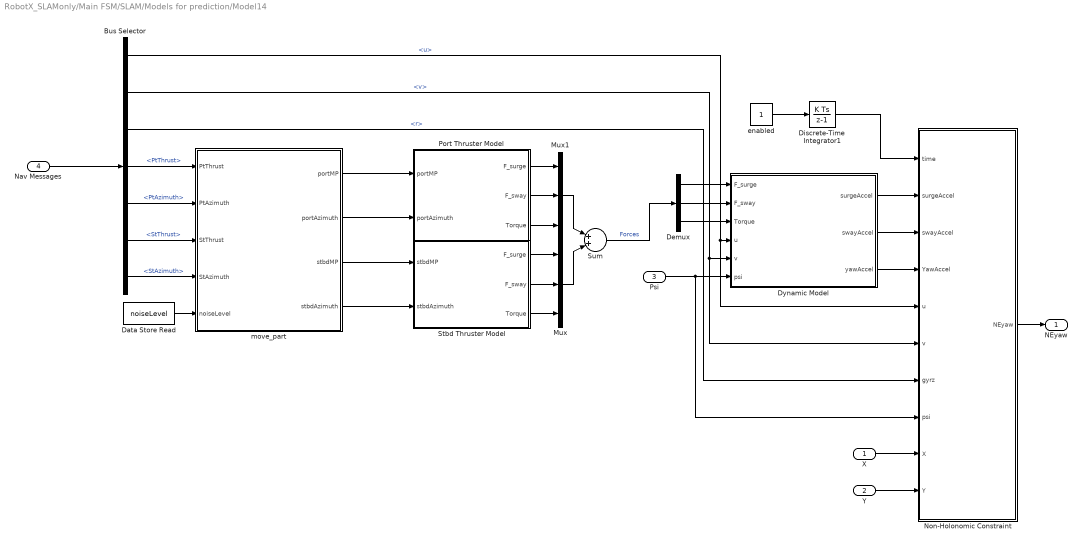
== system RobotX_SLAMonly/Main FSM/SLAM/Models for prediction/Model14 ==
  X : Inport
  Y : Inport  Port=2
  Psi : Inport  Port=3
  Nav Messages : Inport  Port=4
  Bus Selector : BusSelector  OutputSignals=Velocity.u,Velocity.v,Velocity.r,Port.PtThrust,Port.PtAzimuth,Stbd.StThrust,Stbd.StAzimuth
  Data Store Read : DataStoreRead  DataStoreName=noiseLevel
  Demux : Demux  Outputs=3
  Discrete-Time Integrator1 : DiscreteIntegrator  SampleTime=-1  ICPrevOutput=DiscIntNeverNeededParam  ICPrevScaledInput=DiscIntNeverNeededParam
  Dynamic Model : MATLAB Function  TreatAsAtomicUnit=on
  Mux : Mux  Inputs=3
  Mux1 : Mux  Inputs=3
  Non-Holonomic Constraint : MATLAB Function  TreatAsAtomicUnit=on
  Port Thruster Model : MATLAB Function  TreatAsAtomicUnit=on
  Stbd Thruster Model : MATLAB Function  TreatAsAtomicUnit=on
  Sum : Sum  Inputs=|++|
  enabled : Constant
  move_part : MATLAB Function  TreatAsAtomicUnit=on
  NEyaw : Outport
  wires:
  Sum/1 -> Demux/1  "Forces"
  Bus Selector/2 -> Non-Holonomic Constraint/6(v), Dynamic Model/5(v)  "<v>"
  Bus Selector/1 -> Non-Holonomic Constraint/5(u), Dynamic Model/4(u)  "<u>"
  Psi/1 -> Non-Holonomic Constraint/8(psi), Dynamic Model/6(psi)
  Demux/2 -> Dynamic Model/2(F_sway)
  Demux/3 -> Dynamic Model/3(Torque)
  Demux/1 -> Dynamic Model/1(F_surge)
  Mux/1 -> Sum/2
  Stbd Thruster Model/1(F_surge) -> Mux/1
  Stbd Thruster Model/3(Torque) -> Mux/3
  Stbd Thruster Model/2(F_sway) -> Mux/2
  Mux1/1 -> Sum/1
  Port Thruster Model/2(F_sway) -> Mux1/2
  Port Thruster Model/1(F_surge) -> Mux1/1
  Port Thruster Model/3(Torque) -> Mux1/3
  Dynamic Model/1(surgeAccel) -> Non-Holonomic Constraint/2(surgeAccel)
  Dynamic Model/2(swayAccel) -> Non-Holonomic Constraint/3(swayAccel)
  Dynamic Model/3(yawAccel) -> Non-Holonomic Constraint/4(YawAccel)
  Y/1 -> Non-Holonomic Constraint/10(Y)
  X/1 -> Non-Holonomic Constraint/9(X)
  Bus Selector/3 -> Non-Holonomic Constraint/7(gyrz)  "<r>"
  Non-Holonomic Constraint/1(NEyaw) -> NEyaw/1
  enabled/1 -> Discrete-Time Integrator1/1
  Discrete-Time Integrator1/1 -> Non-Holonomic Constraint/1(time)
  Nav Messages/1 -> Bus Selector/1
  Bus Selector/4 -> move_part/1(PtThrust)  "<PtThrust>"
  Bus Selector/5 -> move_part/2(PtAzimuth)  "<PtAzimuth>"
  Bus Selector/7 -> move_part/4(StAzimuth)  "<StAzimuth>"
  Bus Selector/6 -> move_part/3(StThrust)  "<StThrust>"
  move_part/1(portMP) -> Port Thruster Model/1(portMP)
  move_part/2(portAzimuth) -> Port Thruster Model/2(portAzimuth)
  move_part/3(stbdMP) -> Stbd Thruster Model/1(stbdMP)
  move_part/4(stbdAzimuth) -> Stbd Thruster Model/2(stbdAzimuth)
  Data Store Read/1 -> move_part/5(noiseLevel)

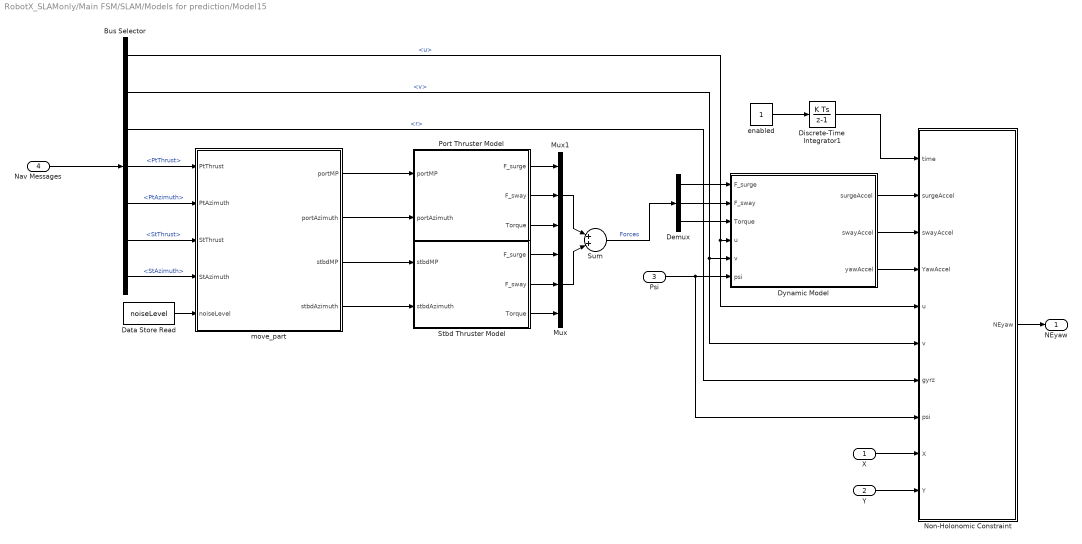
== system RobotX_SLAMonly/Main FSM/SLAM/Models for prediction/Model15 ==
  X : Inport
  Y : Inport  Port=2
  Psi : Inport  Port=3
  Nav Messages : Inport  Port=4
  Bus Selector : BusSelector  OutputSignals=Velocity.u,Velocity.v,Velocity.r,Port.PtThrust,Port.PtAzimuth,Stbd.StThrust,Stbd.StAzimuth
  Data Store Read : DataStoreRead  DataStoreName=noiseLevel
  Demux : Demux  Outputs=3
  Discrete-Time Integrator1 : DiscreteIntegrator  SampleTime=-1  ICPrevOutput=DiscIntNeverNeededParam  ICPrevScaledInput=DiscIntNeverNeededParam
  Dynamic Model : MATLAB Function  TreatAsAtomicUnit=on
  Mux : Mux  Inputs=3
  Mux1 : Mux  Inputs=3
  Non-Holonomic Constraint : MATLAB Function  TreatAsAtomicUnit=on
  Port Thruster Model : MATLAB Function  TreatAsAtomicUnit=on
  Stbd Thruster Model : MATLAB Function  TreatAsAtomicUnit=on
  Sum : Sum  Inputs=|++|
  enabled : Constant
  move_part : MATLAB Function  TreatAsAtomicUnit=on
  NEyaw : Outport
  wires:
  Sum/1 -> Demux/1  "Forces"
  Bus Selector/2 -> Non-Holonomic Constraint/6(v), Dynamic Model/5(v)  "<v>"
  Bus Selector/1 -> Non-Holonomic Constraint/5(u), Dynamic Model/4(u)  "<u>"
  Psi/1 -> Non-Holonomic Constraint/8(psi), Dynamic Model/6(psi)
  Demux/2 -> Dynamic Model/2(F_sway)
  Demux/3 -> Dynamic Model/3(Torque)
  Demux/1 -> Dynamic Model/1(F_surge)
  Mux/1 -> Sum/2
  Stbd Thruster Model/1(F_surge) -> Mux/1
  Stbd Thruster Model/3(Torque) -> Mux/3
  Stbd Thruster Model/2(F_sway) -> Mux/2
  Mux1/1 -> Sum/1
  Port Thruster Model/2(F_sway) -> Mux1/2
  Port Thruster Model/1(F_surge) -> Mux1/1
  Port Thruster Model/3(Torque) -> Mux1/3
  Dynamic Model/1(surgeAccel) -> Non-Holonomic Constraint/2(surgeAccel)
  Dynamic Model/2(swayAccel) -> Non-Holonomic Constraint/3(swayAccel)
  Dynamic Model/3(yawAccel) -> Non-Holonomic Constraint/4(YawAccel)
  Y/1 -> Non-Holonomic Constraint/10(Y)
  X/1 -> Non-Holonomic Constraint/9(X)
  Bus Selector/3 -> Non-Holonomic Constraint/7(gyrz)  "<r>"
  Non-Holonomic Constraint/1(NEyaw) -> NEyaw/1
  enabled/1 -> Discrete-Time Integrator1/1
  Discrete-Time Integrator1/1 -> Non-Holonomic Constraint/1(time)
  Nav Messages/1 -> Bus Selector/1
  Bus Selector/4 -> move_part/1(PtThrust)  "<PtThrust>"
  Bus Selector/5 -> move_part/2(PtAzimuth)  "<PtAzimuth>"
  Bus Selector/7 -> move_part/4(StAzimuth)  "<StAzimuth>"
  Bus Selector/6 -> move_part/3(StThrust)  "<StThrust>"
  move_part/1(portMP) -> Port Thruster Model/1(portMP)
  move_part/2(portAzimuth) -> Port Thruster Model/2(portAzimuth)
  move_part/3(stbdMP) -> Stbd Thruster Model/1(stbdMP)
  move_part/4(stbdAzimuth) -> Stbd Thruster Model/2(stbdAzimuth)
  Data Store Read/1 -> move_part/5(noiseLevel)
